simulink model "Demo_PreScanCarSim3D_ExtFMU_cs"  (Simulink 8.6)
settings: Solver=ode5  SolverMode=SingleTasking  StartTime=0.0  StopTime=68  FixedStep=1/1000  RelTol=1e-3
PreLoadFcn:
  | mbxruntime.callbacks.PreLoadFcn(bdroot);
  | check_NUTS_defined;
  | 
  | assignin('base',['model_closed_' bdroot],false);
PostLoadFcn:
  | mbxruntime.callbacks.PostLoadFcn(bdroot);
InitFcn:
  | mbxruntime.callbacks.InitFcn(bdroot);
StartFcn:
  | mbxruntime.callbacks.StartFcn(bdroot);
StopFcn:
  | mbxruntime.callbacks.StopFcn(bdroot);
undefined symbols (not defined in the file): DiscIntNeverNeededParam, mbxruntime, tabledata, warningInitialVelocity, x0, x_ini_VRML, y_ini_VRML, z_ini_VRML
libraries: PreScanSimulinkLibrary x15, simulink_extras x8, simulink x5, PreScanCarSimLibrary x1
(part 7 of 11)

== system Demo_PreScanCarSim3D_ExtFMU_cs/VISUMatrixSign_HighwayOverhang_1/ENABLED/Actuator ==
  VISUMatrixSign_HighwayOverhang_1 : Inport  Tag=inport/VisuMatrixSign  SampleTime=50/1000  BusOutputAsStruct=on
  DemuxVisuMatrixSign : Demux
  visu_MatrixSign_1 : S-Function  FunctionName=sfun_ResourceNameSelector  Parameters=mbxruntime.parameters.convert(UniqueID), mbxruntime.parameters.convert(ResourceList), mbxruntime.parameters.convert(PivotName),tabledata, TimeStep  SFunctionDeploymentMode=off  EnableBusSupport=off  mask(PreScan Sink Block: VisuMatrixSign){UniqueID=1876, ResourceList={'3' 'InformationSign\MatrixSign_Empty.png' '4' 'InformationSign\MatrixSign_End.png' '5' 'InformationSign\MatrixSign_GreenArrow.png' '6' 'InformationSign\MatrixSign_RedCross.png' '7' 'InformationSign\MatrixSign_Speed_50.png' '8' 'InformationSign\MatrixSign_Speed_70.png' '9' 'InformationSign\MatrixSign_Speed_90.png' '10' 'InformationSign\MatrixSign_Speed_120.png' '11' 'InformationSign\MatrixSign_Speed_130.png' '12' 'InformationSign\information.png' '13' 'InformationSign\TASS-international-logo.bmp' }, PivotName=/child:name=hcn/child:name=MatrixSign_1/trafficSignElement, TimeStep=50/1000}
      mask prompts: UniqueID "Parent Unique Identifier (auto-generated)"; ResourceList "Resource List (auto-generated)"; PivotName "Name of pivot (auto-generated)"; TimeStep "Simulink time step"
      mask help:
      | The VisuMatrixSign block provides a way to adapt the texture of the plates connected to an overhang, based on Resource IDs of the texture files.
      |
      | For more information, please click Help.
      mask init:
      | [tabledata] = mbxruntime.parameters.table(UniqueID,ResourceList,PivotName);
      mask Help: eval('openHelp(733)')
      mask Display: image(imread('HighwaySpeedMatrix.png'))
  visu_MatrixSign_2 : S-Function  FunctionName=sfun_ResourceNameSelector  Parameters=mbxruntime.parameters.convert(UniqueID), mbxruntime.parameters.convert(ResourceList), mbxruntime.parameters.convert(PivotName),tabledata, TimeStep  SFunctionDeploymentMode=off  EnableBusSupport=off  mask(PreScan Sink Block: VisuMatrixSign){UniqueID=1876, ResourceList={'3' 'InformationSign\MatrixSign_Empty.png' '4' 'InformationSign\MatrixSign_End.png' '5' 'InformationSign\MatrixSign_GreenArrow.png' '6' 'InformationSign\MatrixSign_RedCross.png' '7' 'InformationSign\MatrixSign_Speed_50.png' '8' 'InformationSign\MatrixSign_Speed_70.png' '9' 'InformationSign\MatrixSign_Speed_90.png' '10' 'InformationSign\MatrixSign_Speed_120.png' '11' 'InformationSign\MatrixSign_Speed_130.png' '12' 'InformationSign\information.png' '13' 'InformationSign\TASS-international-logo.bmp' }, PivotName=/child:name=hcn/child:name=MatrixSign_2/trafficSignElement, TimeStep=50/1000}
      mask prompts: UniqueID "Parent Unique Identifier (auto-generated)"; ResourceList "Resource List (auto-generated)"; PivotName "Name of pivot (auto-generated)"; TimeStep "Simulink time step"
      mask help:
      | The VisuMatrixSign block provides a way to adapt the texture of the plates connected to an overhang, based on Resource IDs of the texture files.
      |
      | For more information, please click Help.
      mask init:
      | [tabledata] = mbxruntime.parameters.table(UniqueID,ResourceList,PivotName);
      mask Help: eval('openHelp(733)')
      mask Display: image(imread('HighwaySpeedMatrix.png'))
  visu_MatrixSign_3 : S-Function  FunctionName=sfun_ResourceNameSelector  Parameters=mbxruntime.parameters.convert(UniqueID), mbxruntime.parameters.convert(ResourceList), mbxruntime.parameters.convert(PivotName),tabledata, TimeStep  SFunctionDeploymentMode=off  EnableBusSupport=off  mask(PreScan Sink Block: VisuMatrixSign){UniqueID=1876, ResourceList={'3' 'InformationSign\MatrixSign_Empty.png' '4' 'InformationSign\MatrixSign_End.png' '5' 'InformationSign\MatrixSign_GreenArrow.png' '6' 'InformationSign\MatrixSign_RedCross.png' '7' 'InformationSign\MatrixSign_Speed_50.png' '8' 'InformationSign\MatrixSign_Speed_70.png' '9' 'InformationSign\MatrixSign_Speed_90.png' '10' 'InformationSign\MatrixSign_Speed_120.png' '11' 'InformationSign\MatrixSign_Speed_130.png' '12' 'InformationSign\information.png' '13' 'InformationSign\TASS-international-logo.bmp' }, PivotName=/child:name=hcn/child:name=MatrixSign_3/trafficSignElement, TimeStep=50/1000}
      mask prompts: UniqueID "Parent Unique Identifier (auto-generated)"; ResourceList "Resource List (auto-generated)"; PivotName "Name of pivot (auto-generated)"; TimeStep "Simulink time step"
      mask help:
      | The VisuMatrixSign block provides a way to adapt the texture of the plates connected to an overhang, based on Resource IDs of the texture files.
      |
      | For more information, please click Help.
      mask init:
      | [tabledata] = mbxruntime.parameters.table(UniqueID,ResourceList,PivotName);
      mask Help: eval('openHelp(733)')
      mask Display: image(imread('HighwaySpeedMatrix.png'))
  visu_MatrixSign_4 : S-Function  FunctionName=sfun_ResourceNameSelector  Parameters=mbxruntime.parameters.convert(UniqueID), mbxruntime.parameters.convert(ResourceList), mbxruntime.parameters.convert(PivotName),tabledata, TimeStep  SFunctionDeploymentMode=off  EnableBusSupport=off  mask(PreScan Sink Block: VisuMatrixSign){UniqueID=1876, ResourceList={'3' 'InformationSign\MatrixSign_Empty.png' '4' 'InformationSign\MatrixSign_End.png' '5' 'InformationSign\MatrixSign_GreenArrow.png' '6' 'InformationSign\MatrixSign_RedCross.png' '7' 'InformationSign\MatrixSign_Speed_50.png' '8' 'InformationSign\MatrixSign_Speed_70.png' '9' 'InformationSign\MatrixSign_Speed_90.png' '10' 'InformationSign\MatrixSign_Speed_120.png' '11' 'InformationSign\MatrixSign_Speed_130.png' '12' 'InformationSign\information.png' '13' 'InformationSign\TASS-international-logo.bmp' }, PivotName=/child:name=hcn/child:name=MatrixSign_4/trafficSignElement, TimeStep=50/1000}
      mask prompts: UniqueID "Parent Unique Identifier (auto-generated)"; ResourceList "Resource List (auto-generated)"; PivotName "Name of pivot (auto-generated)"; TimeStep "Simulink time step"
      mask help:
      | The VisuMatrixSign block provides a way to adapt the texture of the plates connected to an overhang, based on Resource IDs of the texture files.
      |
      | For more information, please click Help.
      mask init:
      | [tabledata] = mbxruntime.parameters.table(UniqueID,ResourceList,PivotName);
      mask Help: eval('openHelp(733)')
      mask Display: image(imread('HighwaySpeedMatrix.png'))
  wires:
  VISUMatrixSign_HighwayOverhang_1/1 -> DemuxVisuMatrixSign/1
  DemuxVisuMatrixSign/1 -> visu_MatrixSign_1/1
  DemuxVisuMatrixSign/2 -> visu_MatrixSign_2/1
  DemuxVisuMatrixSign/3 -> visu_MatrixSign_3/1
  DemuxVisuMatrixSign/4 -> visu_MatrixSign_4/1

== system Demo_PreScanCarSim3D_ExtFMU_cs/VISUMatrixSign_HighwayOverhang_2/ENABLED/Actuator ==
  VISUMatrixSign_HighwayOverhang_2 : Inport  Tag=inport/VisuMatrixSign  SampleTime=50/1000  BusOutputAsStruct=on
  DemuxVisuMatrixSign : Demux  Outputs=3
  visu_MatrixSign_5 : S-Function  FunctionName=sfun_ResourceNameSelector  Parameters=mbxruntime.parameters.convert(UniqueID), mbxruntime.parameters.convert(ResourceList), mbxruntime.parameters.convert(PivotName),tabledata, TimeStep  SFunctionDeploymentMode=off  EnableBusSupport=off  mask(PreScan Sink Block: VisuMatrixSign){UniqueID=1877, ResourceList={'3' 'InformationSign\MatrixSign_Empty.png' '4' 'InformationSign\MatrixSign_End.png' '5' 'InformationSign\MatrixSign_GreenArrow.png' '6' 'InformationSign\MatrixSign_RedCross.png' '7' 'InformationSign\MatrixSign_Speed_50.png' '8' 'InformationSign\MatrixSign_Speed_70.png' '9' 'InformationSign\MatrixSign_Speed_90.png' '10' 'InformationSign\MatrixSign_Speed_120.png' '11' 'InformationSign\MatrixSign_Speed_130.png' '12' 'InformationSign\information.png' '13' 'InformationSign\TASS-international-logo.bmp' }, PivotName=/child:name=hcn/child:name=MatrixSign_5/trafficSignElement, TimeStep=50/1000}
      mask prompts: UniqueID "Parent Unique Identifier (auto-generated)"; ResourceList "Resource List (auto-generated)"; PivotName "Name of pivot (auto-generated)"; TimeStep "Simulink time step"
      mask help:
      | The VisuMatrixSign block provides a way to adapt the texture of the plates connected to an overhang, based on Resource IDs of the texture files.
      |
      | For more information, please click Help.
      mask init:
      | [tabledata] = mbxruntime.parameters.table(UniqueID,ResourceList,PivotName);
      mask Help: eval('openHelp(733)')
      mask Display: image(imread('HighwaySpeedMatrix.png'))
  visu_MatrixSign_6 : S-Function  FunctionName=sfun_ResourceNameSelector  Parameters=mbxruntime.parameters.convert(UniqueID), mbxruntime.parameters.convert(ResourceList), mbxruntime.parameters.convert(PivotName),tabledata, TimeStep  SFunctionDeploymentMode=off  EnableBusSupport=off  mask(PreScan Sink Block: VisuMatrixSign){UniqueID=1877, ResourceList={'3' 'InformationSign\MatrixSign_Empty.png' '4' 'InformationSign\MatrixSign_End.png' '5' 'InformationSign\MatrixSign_GreenArrow.png' '6' 'InformationSign\MatrixSign_RedCross.png' '7' 'InformationSign\MatrixSign_Speed_50.png' '8' 'InformationSign\MatrixSign_Speed_70.png' '9' 'InformationSign\MatrixSign_Speed_90.png' '10' 'InformationSign\MatrixSign_Speed_120.png' '11' 'InformationSign\MatrixSign_Speed_130.png' '12' 'InformationSign\information.png' '13' 'InformationSign\TASS-international-logo.bmp' }, PivotName=/child:name=hcn/child:name=MatrixSign_6/trafficSignElement, TimeStep=50/1000}
      mask prompts: UniqueID "Parent Unique Identifier (auto-generated)"; ResourceList "Resource List (auto-generated)"; PivotName "Name of pivot (auto-generated)"; TimeStep "Simulink time step"
      mask help:
      | The VisuMatrixSign block provides a way to adapt the texture of the plates connected to an overhang, based on Resource IDs of the texture files.
      |
      | For more information, please click Help.
      mask init:
      | [tabledata] = mbxruntime.parameters.table(UniqueID,ResourceList,PivotName);
      mask Help: eval('openHelp(733)')
      mask Display: image(imread('HighwaySpeedMatrix.png'))
  visu_MatrixSign_7 : S-Function  FunctionName=sfun_ResourceNameSelector  Parameters=mbxruntime.parameters.convert(UniqueID), mbxruntime.parameters.convert(ResourceList), mbxruntime.parameters.convert(PivotName),tabledata, TimeStep  SFunctionDeploymentMode=off  EnableBusSupport=off  mask(PreScan Sink Block: VisuMatrixSign){UniqueID=1877, ResourceList={'3' 'InformationSign\MatrixSign_Empty.png' '4' 'InformationSign\MatrixSign_End.png' '5' 'InformationSign\MatrixSign_GreenArrow.png' '6' 'InformationSign\MatrixSign_RedCross.png' '7' 'InformationSign\MatrixSign_Speed_50.png' '8' 'InformationSign\MatrixSign_Speed_70.png' '9' 'InformationSign\MatrixSign_Speed_90.png' '10' 'InformationSign\MatrixSign_Speed_120.png' '11' 'InformationSign\MatrixSign_Speed_130.png' '12' 'InformationSign\information.png' '13' 'InformationSign\TASS-international-logo.bmp' }, PivotName=/child:name=hcn/child:name=MatrixSign_7/trafficSignElement, TimeStep=50/1000}
      mask prompts: UniqueID "Parent Unique Identifier (auto-generated)"; ResourceList "Resource List (auto-generated)"; PivotName "Name of pivot (auto-generated)"; TimeStep "Simulink time step"
      mask help:
      | The VisuMatrixSign block provides a way to adapt the texture of the plates connected to an overhang, based on Resource IDs of the texture files.
      |
      | For more information, please click Help.
      mask init:
      | [tabledata] = mbxruntime.parameters.table(UniqueID,ResourceList,PivotName);
      mask Help: eval('openHelp(733)')
      mask Display: image(imread('HighwaySpeedMatrix.png'))
  wires:
  VISUMatrixSign_HighwayOverhang_2/1 -> DemuxVisuMatrixSign/1
  DemuxVisuMatrixSign/1 -> visu_MatrixSign_5/1
  DemuxVisuMatrixSign/2 -> visu_MatrixSign_6/1
  DemuxVisuMatrixSign/3 -> visu_MatrixSign_7/1

== system Demo_PreScanCarSim3D_ExtFMU_cs/VISUMatrixSign_HighwayOverhang_3/ENABLED/Actuator ==
  VISUMatrixSign_HighwayOverhang_3 : Inport  Tag=inport/VisuMatrixSign  SampleTime=50/1000  BusOutputAsStruct=on
  DemuxVisuMatrixSign : Demux  Outputs=3
  visu_MatrixSign_10 : S-Function  FunctionName=sfun_ResourceNameSelector  Parameters=mbxruntime.parameters.convert(UniqueID), mbxruntime.parameters.convert(ResourceList), mbxruntime.parameters.convert(PivotName),tabledata, TimeStep  SFunctionDeploymentMode=off  EnableBusSupport=off  mask(PreScan Sink Block: VisuMatrixSign){UniqueID=1890, ResourceList={'3' 'InformationSign\MatrixSign_Empty.png' '4' 'InformationSign\MatrixSign_End.png' '5' 'InformationSign\MatrixSign_GreenArrow.png' '6' 'InformationSign\MatrixSign_RedCross.png' '7' 'InformationSign\MatrixSign_Speed_50.png' '8' 'InformationSign\MatrixSign_Speed_70.png' '9' 'InformationSign\MatrixSign_Speed_90.png' '10' 'InformationSign\MatrixSign_Speed_120.png' '11' 'InformationSign\MatrixSign_Speed_130.png' '12' 'InformationSign\information.png' '13' 'InformationSign\TASS-international-logo.bmp' }, PivotName=/child:name=hcn/child:name=MatrixSign_10/trafficSignElement, TimeStep=50/1000}
      mask prompts: UniqueID "Parent Unique Identifier (auto-generated)"; ResourceList "Resource List (auto-generated)"; PivotName "Name of pivot (auto-generated)"; TimeStep "Simulink time step"
      mask help:
      | The VisuMatrixSign block provides a way to adapt the texture of the plates connected to an overhang, based on Resource IDs of the texture files.
      |
      | For more information, please click Help.
      mask init:
      | [tabledata] = mbxruntime.parameters.table(UniqueID,ResourceList,PivotName);
      mask Help: eval('openHelp(733)')
      mask Display: image(imread('HighwaySpeedMatrix.png'))
  visu_MatrixSign_11 : S-Function  FunctionName=sfun_ResourceNameSelector  Parameters=mbxruntime.parameters.convert(UniqueID), mbxruntime.parameters.convert(ResourceList), mbxruntime.parameters.convert(PivotName),tabledata, TimeStep  SFunctionDeploymentMode=off  EnableBusSupport=off  mask(PreScan Sink Block: VisuMatrixSign){UniqueID=1890, ResourceList={'3' 'InformationSign\MatrixSign_Empty.png' '4' 'InformationSign\MatrixSign_End.png' '5' 'InformationSign\MatrixSign_GreenArrow.png' '6' 'InformationSign\MatrixSign_RedCross.png' '7' 'InformationSign\MatrixSign_Speed_50.png' '8' 'InformationSign\MatrixSign_Speed_70.png' '9' 'InformationSign\MatrixSign_Speed_90.png' '10' 'InformationSign\MatrixSign_Speed_120.png' '11' 'InformationSign\MatrixSign_Speed_130.png' '12' 'InformationSign\information.png' '13' 'InformationSign\TASS-international-logo.bmp' }, PivotName=/child:name=hcn/child:name=MatrixSign_11/trafficSignElement, TimeStep=50/1000}
      mask prompts: UniqueID "Parent Unique Identifier (auto-generated)"; ResourceList "Resource List (auto-generated)"; PivotName "Name of pivot (auto-generated)"; TimeStep "Simulink time step"
      mask help:
      | The VisuMatrixSign block provides a way to adapt the texture of the plates connected to an overhang, based on Resource IDs of the texture files.
      |
      | For more information, please click Help.
      mask init:
      | [tabledata] = mbxruntime.parameters.table(UniqueID,ResourceList,PivotName);
      mask Help: eval('openHelp(733)')
      mask Display: image(imread('HighwaySpeedMatrix.png'))
  visu_MatrixSign_12 : S-Function  FunctionName=sfun_ResourceNameSelector  Parameters=mbxruntime.parameters.convert(UniqueID), mbxruntime.parameters.convert(ResourceList), mbxruntime.parameters.convert(PivotName),tabledata, TimeStep  SFunctionDeploymentMode=off  EnableBusSupport=off  mask(PreScan Sink Block: VisuMatrixSign){UniqueID=1890, ResourceList={'3' 'InformationSign\MatrixSign_Empty.png' '4' 'InformationSign\MatrixSign_End.png' '5' 'InformationSign\MatrixSign_GreenArrow.png' '6' 'InformationSign\MatrixSign_RedCross.png' '7' 'InformationSign\MatrixSign_Speed_50.png' '8' 'InformationSign\MatrixSign_Speed_70.png' '9' 'InformationSign\MatrixSign_Speed_90.png' '10' 'InformationSign\MatrixSign_Speed_120.png' '11' 'InformationSign\MatrixSign_Speed_130.png' '12' 'InformationSign\information.png' '13' 'InformationSign\TASS-international-logo.bmp' }, PivotName=/child:name=hcn/child:name=MatrixSign_12/trafficSignElement, TimeStep=50/1000}
      mask prompts: UniqueID "Parent Unique Identifier (auto-generated)"; ResourceList "Resource List (auto-generated)"; PivotName "Name of pivot (auto-generated)"; TimeStep "Simulink time step"
      mask help:
      | The VisuMatrixSign block provides a way to adapt the texture of the plates connected to an overhang, based on Resource IDs of the texture files.
      |
      | For more information, please click Help.
      mask init:
      | [tabledata] = mbxruntime.parameters.table(UniqueID,ResourceList,PivotName);
      mask Help: eval('openHelp(733)')
      mask Display: image(imread('HighwaySpeedMatrix.png'))
  wires:
  VISUMatrixSign_HighwayOverhang_3/1 -> DemuxVisuMatrixSign/1
  DemuxVisuMatrixSign/1 -> visu_MatrixSign_10/1
  DemuxVisuMatrixSign/2 -> visu_MatrixSign_11/1
  DemuxVisuMatrixSign/3 -> visu_MatrixSign_12/1

== system Demo_PreScanCarSim3D_ExtFMU_cs/VISUMatrixSign_HighwayOverhang_5/ENABLED/Actuator ==
  VISUMatrixSign_HighwayOverhang_5 : Inport  Tag=inport/VisuMatrixSign  SampleTime=50/1000  BusOutputAsStruct=on
  DemuxVisuMatrixSign : Demux  Outputs=3
  visu_MatrixSign_18 : S-Function  FunctionName=sfun_ResourceNameSelector  Parameters=mbxruntime.parameters.convert(UniqueID), mbxruntime.parameters.convert(ResourceList), mbxruntime.parameters.convert(PivotName),tabledata, TimeStep  SFunctionDeploymentMode=off  EnableBusSupport=off  mask(PreScan Sink Block: VisuMatrixSign){UniqueID=1909, ResourceList={'3' 'InformationSign\MatrixSign_Empty.png' '4' 'InformationSign\MatrixSign_End.png' '5' 'InformationSign\MatrixSign_GreenArrow.png' '6' 'InformationSign\MatrixSign_RedCross.png' '7' 'InformationSign\MatrixSign_Speed_50.png' '8' 'InformationSign\MatrixSign_Speed_70.png' '9' 'InformationSign\MatrixSign_Speed_90.png' '10' 'InformationSign\MatrixSign_Speed_120.png' '11' 'InformationSign\MatrixSign_Speed_130.png' '12' 'InformationSign\information.png' '13' 'InformationSign\TASS-international-logo.bmp' }, PivotName=/child:name=hcn/child:name=MatrixSign_18/trafficSignElement, TimeStep=50/1000}
      mask prompts: UniqueID "Parent Unique Identifier (auto-generated)"; ResourceList "Resource List (auto-generated)"; PivotName "Name of pivot (auto-generated)"; TimeStep "Simulink time step"
      mask help:
      | The VisuMatrixSign block provides a way to adapt the texture of the plates connected to an overhang, based on Resource IDs of the texture files.
      |
      | For more information, please click Help.
      mask init:
      | [tabledata] = mbxruntime.parameters.table(UniqueID,ResourceList,PivotName);
      mask Help: eval('openHelp(733)')
      mask Display: image(imread('HighwaySpeedMatrix.png'))
  visu_MatrixSign_19 : S-Function  FunctionName=sfun_ResourceNameSelector  Parameters=mbxruntime.parameters.convert(UniqueID), mbxruntime.parameters.convert(ResourceList), mbxruntime.parameters.convert(PivotName),tabledata, TimeStep  SFunctionDeploymentMode=off  EnableBusSupport=off  mask(PreScan Sink Block: VisuMatrixSign){UniqueID=1909, ResourceList={'3' 'InformationSign\MatrixSign_Empty.png' '4' 'InformationSign\MatrixSign_End.png' '5' 'InformationSign\MatrixSign_GreenArrow.png' '6' 'InformationSign\MatrixSign_RedCross.png' '7' 'InformationSign\MatrixSign_Speed_50.png' '8' 'InformationSign\MatrixSign_Speed_70.png' '9' 'InformationSign\MatrixSign_Speed_90.png' '10' 'InformationSign\MatrixSign_Speed_120.png' '11' 'InformationSign\MatrixSign_Speed_130.png' '12' 'InformationSign\information.png' '13' 'InformationSign\TASS-international-logo.bmp' }, PivotName=/child:name=hcn/child:name=MatrixSign_19/trafficSignElement, TimeStep=50/1000}
      mask prompts: UniqueID "Parent Unique Identifier (auto-generated)"; ResourceList "Resource List (auto-generated)"; PivotName "Name of pivot (auto-generated)"; TimeStep "Simulink time step"
      mask help:
      | The VisuMatrixSign block provides a way to adapt the texture of the plates connected to an overhang, based on Resource IDs of the texture files.
      |
      | For more information, please click Help.
      mask init:
      | [tabledata] = mbxruntime.parameters.table(UniqueID,ResourceList,PivotName);
      mask Help: eval('openHelp(733)')
      mask Display: image(imread('HighwaySpeedMatrix.png'))
  visu_MatrixSign_20 : S-Function  FunctionName=sfun_ResourceNameSelector  Parameters=mbxruntime.parameters.convert(UniqueID), mbxruntime.parameters.convert(ResourceList), mbxruntime.parameters.convert(PivotName),tabledata, TimeStep  SFunctionDeploymentMode=off  EnableBusSupport=off  mask(PreScan Sink Block: VisuMatrixSign){UniqueID=1909, ResourceList={'3' 'InformationSign\MatrixSign_Empty.png' '4' 'InformationSign\MatrixSign_End.png' '5' 'InformationSign\MatrixSign_GreenArrow.png' '6' 'InformationSign\MatrixSign_RedCross.png' '7' 'InformationSign\MatrixSign_Speed_50.png' '8' 'InformationSign\MatrixSign_Speed_70.png' '9' 'InformationSign\MatrixSign_Speed_90.png' '10' 'InformationSign\MatrixSign_Speed_120.png' '11' 'InformationSign\MatrixSign_Speed_130.png' '12' 'InformationSign\information.png' '13' 'InformationSign\TASS-international-logo.bmp' }, PivotName=/child:name=hcn/child:name=MatrixSign_20/trafficSignElement, TimeStep=50/1000}
      mask prompts: UniqueID "Parent Unique Identifier (auto-generated)"; ResourceList "Resource List (auto-generated)"; PivotName "Name of pivot (auto-generated)"; TimeStep "Simulink time step"
      mask help:
      | The VisuMatrixSign block provides a way to adapt the texture of the plates connected to an overhang, based on Resource IDs of the texture files.
      |
      | For more information, please click Help.
      mask init:
      | [tabledata] = mbxruntime.parameters.table(UniqueID,ResourceList,PivotName);
      mask Help: eval('openHelp(733)')
      mask Display: image(imread('HighwaySpeedMatrix.png'))
  wires:
  VISUMatrixSign_HighwayOverhang_5/1 -> DemuxVisuMatrixSign/1
  DemuxVisuMatrixSign/1 -> visu_MatrixSign_18/1
  DemuxVisuMatrixSign/2 -> visu_MatrixSign_19/1
  DemuxVisuMatrixSign/3 -> visu_MatrixSign_20/1

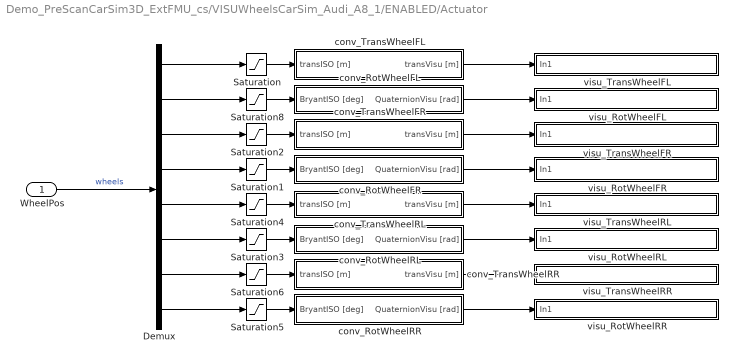
== system Demo_PreScanCarSim3D_ExtFMU_cs/VISUWheelsCarSim_Audi_A8_1/ENABLED/Actuator ==
  WheelPos : Inport
  Demux : Demux  Outputs=[3 3 3 3 3 3 3 3]
  Saturation{,2,4,6} (4 alike) : Saturate  UpperLimit=[0.2 0.2 0.5]  LowerLimit=[-0.2 -0.2 -0.5]
  Saturation{1,3,5,8} (4 alike) : Saturate  UpperLimit=[30 inf 30]  LowerLimit=[-30 -inf -30]
  conv_RotWheelFL : Subsystem
  conv_RotWheelFR : Subsystem
  conv_RotWheelRL : Subsystem
  conv_RotWheelRR : Subsystem
  conv_TransWheelFL : Subsystem  mask(Translation node configuration){tp=Front-Left Wheel, gains=off, Gain_xISO=1, Gain_yISO=1, Gain_zISO=1}
      mask prompts: tp "Type"; gains "Edit scaling factors?"; Gain_xISO "Scaling factor in x-direction (ISO-convention)"; Gain_yISO "Scaling factor in y-direction (ISO-convention)"; Gain_zISO "Scaling factor in z-direction (ISO-convention)"
      mask init:
      | [x_ini_VRML,y_ini_VRML,z_ini_VRML]=Visu_ini_param('Audi_A8',tp);
      mask TypeOptions tp: Front-Left Wheel | Front-Right Wheel | Rear-Left Wheel | Rear-Right Wheel | Left Seat | Right Seat
      mask Callback gains:
      | if strcmp(get_param(gcb, 'gains'),'on')
      |     set_param(gcb,'MaskVisibilities',{'on','on','on','on','on'})
      | else
      |     set_param(gcb,'MaskVisibilities',{'on','on','off','off','off'})
      | end
  conv_TransWheelFR : Subsystem  mask(Translation node configuration){tp=Front-Right Wheel, gains=off, Gain_xISO=1, Gain_yISO=1, Gain_zISO=1}
      mask prompts: tp "Type"; gains "Edit scaling factors?"; Gain_xISO "Scaling factor in x-direction (ISO-convention)"; Gain_yISO "Scaling factor in y-direction (ISO-convention)"; Gain_zISO "Scaling factor in z-direction (ISO-convention)"
      mask init:
      | [x_ini_VRML,y_ini_VRML,z_ini_VRML]=Visu_ini_param('Audi_A8',tp);
      mask TypeOptions tp: Front-Left Wheel | Front-Right Wheel | Rear-Left Wheel | Rear-Right Wheel | Left Seat | Right Seat
      mask Callback gains:
      | if strcmp(get_param(gcb, 'gains'),'on')
      |     set_param(gcb,'MaskVisibilities',{'on','on','on','on','on'})
      | else
      |     set_param(gcb,'MaskVisibilities',{'on','on','off','off','off'})
      | end
  conv_TransWheelRL : Subsystem  mask(Translation node configuration){tp=Rear-Left Wheel, gains=off, Gain_xISO=1, Gain_yISO=1, Gain_zISO=1}
      mask prompts: tp "Type"; gains "Edit scaling factors?"; Gain_xISO "Scaling factor in x-direction (ISO-convention)"; Gain_yISO "Scaling factor in y-direction (ISO-convention)"; Gain_zISO "Scaling factor in z-direction (ISO-convention)"
      mask init:
      | [x_ini_VRML,y_ini_VRML,z_ini_VRML]=Visu_ini_param('Audi_A8',tp);
      mask TypeOptions tp: Front-Left Wheel | Front-Right Wheel | Rear-Left Wheel | Rear-Right Wheel | Left Seat | Right Seat
      mask Callback gains:
      | if strcmp(get_param(gcb, 'gains'),'on')
      |     set_param(gcb,'MaskVisibilities',{'on','on','on','on','on'})
      | else
      |     set_param(gcb,'MaskVisibilities',{'on','on','off','off','off'})
      | end
  conv_TransWheelRR : Subsystem  mask(Translation node configuration){tp=Rear-Right Wheel, gains=off, Gain_xISO=1, Gain_yISO=1, Gain_zISO=1}
      mask prompts: tp "Type"; gains "Edit scaling factors?"; Gain_xISO "Scaling factor in x-direction (ISO-convention)"; Gain_yISO "Scaling factor in y-direction (ISO-convention)"; Gain_zISO "Scaling factor in z-direction (ISO-convention)"
      mask init:
      | [x_ini_VRML,y_ini_VRML,z_ini_VRML]=Visu_ini_param('Audi_A8',tp);
      mask TypeOptions tp: Front-Left Wheel | Front-Right Wheel | Rear-Left Wheel | Rear-Right Wheel | Left Seat | Right Seat
      mask Callback gains:
      | if strcmp(get_param(gcb, 'gains'),'on')
      |     set_param(gcb,'MaskVisibilities',{'on','on','on','on','on'})
      | else
      |     set_param(gcb,'MaskVisibilities',{'on','on','off','off','off'})
      | end
  visu_RotWheelFL : Subsystem  mask(AxisAngleActuator){UniqueID=UniqueID, Object3DID=[ObjectName '.WheelFL'], TimeStep=TimeStep}
      mask prompts: UniqueID "Auto-Assigned: Unique ID"; Object3DID "Auto-Assigned: Child 3D Object ID"; TimeStep "Auto-Assigned: Upload Period [s]"
      mask help: Applies axis angle update to selected child object
      mask Help:
      | Applies axis angle update to selected child object
      | 
      | - UniqueID (double)   : Unique ID of the parent actor
      | - Object3DID (string) : Name of the child 3D object
      mask Display: port_label('input', 1, ['AxisAngle ' Object3DID])
  visu_RotWheelFR : Subsystem  mask(AxisAngleActuator){UniqueID=UniqueID, Object3DID=[ObjectName '.WheelFR'], TimeStep=TimeStep}
      mask prompts: UniqueID "Auto-Assigned: Unique ID"; Object3DID "Auto-Assigned: Child 3D Object ID"; TimeStep "Auto-Assigned: Upload Period [s]"
      mask help: Applies axis angle update to selected child object
      mask Help:
      | Applies axis angle update to selected child object
      | 
      | - UniqueID (double)   : Unique ID of the parent actor
      | - Object3DID (string) : Name of the child 3D object
      mask Display: port_label('input', 1, ['AxisAngle ' Object3DID])
  visu_RotWheelRL : Subsystem  mask(AxisAngleActuator){UniqueID=UniqueID, Object3DID=[ObjectName '.WheelRL'], TimeStep=TimeStep}
      mask prompts: UniqueID "Auto-Assigned: Unique ID"; Object3DID "Auto-Assigned: Child 3D Object ID"; TimeStep "Auto-Assigned: Upload Period [s]"
      mask help: Applies axis angle update to selected child object
      mask Help:
      | Applies axis angle update to selected child object
      | 
      | - UniqueID (double)   : Unique ID of the parent actor
      | - Object3DID (string) : Name of the child 3D object
      mask Display: port_label('input', 1, ['AxisAngle ' Object3DID])
  visu_RotWheelRR : Subsystem  mask(AxisAngleActuator){UniqueID=UniqueID, Object3DID=[ObjectName '.WheelRR'], TimeStep=TimeStep}
      mask prompts: UniqueID "Auto-Assigned: Unique ID"; Object3DID "Auto-Assigned: Child 3D Object ID"; TimeStep "Auto-Assigned: Upload Period [s]"
      mask help: Applies axis angle update to selected child object
      mask Help:
      | Applies axis angle update to selected child object
      | 
      | - UniqueID (double)   : Unique ID of the parent actor
      | - Object3DID (string) : Name of the child 3D object
      mask Display: port_label('input', 1, ['AxisAngle ' Object3DID])
  visu_TransWheelFL : Subsystem  mask(PositionActuator){UniqueID=UniqueID, Object3DID=[ObjectName '.WheelFL'], TimeStep=TimeStep}
      mask prompts: UniqueID "Auto-Assigned: Unique ID"; Object3DID "Auto-Assigned: Child 3D Object ID"; TimeStep "Auto-Assigned: Upload Period [s]"
      mask help: Applies position update to selected child object
      mask Help:
      | Applies position update to selected child object
      | 
      | - UniqueID (double)   : Unique ID of the parent actor
      | - Object3DID (string) : Name of the child 3D object
      mask Display: port_label('input', 1, ['Position ' Object3DID])
  visu_TransWheelFR : Subsystem  mask(PositionActuator){UniqueID=UniqueID, Object3DID=[ObjectName '.WheelFR'], TimeStep=TimeStep}
      mask prompts: UniqueID "Auto-Assigned: Unique ID"; Object3DID "Auto-Assigned: Child 3D Object ID"; TimeStep "Auto-Assigned: Upload Period [s]"
      mask help: Applies position update to selected child object
      mask Help:
      | Applies position update to selected child object
      | 
      | - UniqueID (double)   : Unique ID of the parent actor
      | - Object3DID (string) : Name of the child 3D object
      mask Display: port_label('input', 1, ['Position ' Object3DID])
  visu_TransWheelRL : Subsystem  mask(PositionActuator){UniqueID=UniqueID, Object3DID=[ObjectName '.WheelRL'], TimeStep=TimeStep}
      mask prompts: UniqueID "Auto-Assigned: Unique ID"; Object3DID "Auto-Assigned: Child 3D Object ID"; TimeStep "Auto-Assigned: Upload Period [s]"
      mask help: Applies position update to selected child object
      mask Help:
      | Applies position update to selected child object
      | 
      | - UniqueID (double)   : Unique ID of the parent actor
      | - Object3DID (string) : Name of the child 3D object
      mask Display: port_label('input', 1, ['Position ' Object3DID])
  visu_TransWheelRR : Subsystem  mask(PositionActuator){UniqueID=UniqueID, Object3DID=[ObjectName '.WheelRR'], TimeStep=TimeStep}
      mask prompts: UniqueID "Auto-Assigned: Unique ID"; Object3DID "Auto-Assigned: Child 3D Object ID"; TimeStep "Auto-Assigned: Upload Period [s]"
      mask help: Applies position update to selected child object
      mask Help:
      | Applies position update to selected child object
      | 
      | - UniqueID (double)   : Unique ID of the parent actor
      | - Object3DID (string) : Name of the child 3D object
      mask Display: port_label('input', 1, ['Position ' Object3DID])
  wires:
  WheelPos/1 -> Demux/1  "wheels"
  conv_RotWheelRR/1(QuaternionVisu [rad]) -> visu_RotWheelRR/1(In1)
  conv_RotWheelRL/1(QuaternionVisu [rad]) -> visu_RotWheelRL/1(In1)
  conv_RotWheelFR/1(QuaternionVisu [rad]) -> visu_RotWheelFR/1(In1)
  conv_TransWheelRR/1(transVisu [m]) -> visu_TransWheelRR/1(In1)
  conv_TransWheelRL/1(transVisu [m]) -> visu_TransWheelRL/1(In1)
  conv_TransWheelFR/1(transVisu [m]) -> visu_TransWheelFR/1(In1)
  Saturation/1 -> conv_TransWheelFL/1(transISO [m])
  Saturation8/1 -> conv_RotWheelFL/1(BryantISO [deg])
  Saturation2/1 -> conv_TransWheelFR/1(transISO [m])
  Saturation1/1 -> conv_RotWheelFR/1(BryantISO [deg])
  Saturation4/1 -> conv_TransWheelRL/1(transISO [m])
  Saturation3/1 -> conv_RotWheelRL/1(BryantISO [deg])
  Saturation6/1 -> conv_TransWheelRR/1(transISO [m])
  Saturation5/1 -> conv_RotWheelRR/1(BryantISO [deg])
  Demux/1 -> Saturation/1
  Demux/2 -> Saturation8/1
  Demux/3 -> Saturation2/1
  Demux/4 -> Saturation1/1
  Demux/5 -> Saturation4/1
  Demux/6 -> Saturation3/1
  Demux/7 -> Saturation6/1
  Demux/8 -> Saturation5/1
  conv_TransWheelFL/1(transVisu [m]) -> visu_TransWheelFL/1(In1)
  conv_RotWheelFL/1(QuaternionVisu [rad]) -> visu_RotWheelFL/1(In1)

== system Demo_PreScanCarSim3D_ExtFMU_cs/Audi_A8_1/ENABLED/CarSim_Vehicle/CarSim2PreScanSTATE ==
  CarSim_In : Inport
  D2R : Gain  Gain=pi/180
  Demux : Demux  Outputs=[3 3 3 -1]
  Demux1 : Demux  Outputs=3
  Demux2 : Demux  Outputs=3
  Demux3 : Demux  Outputs=3
  Terminator : Terminator
  Transformation_SprungMassCarSim2PreScan : Subsystem
  km|h_to_m|s : Gain  Gain=1/3.6
  x [m] : Outport
  y [m] : Outport  Port=2
  z [m] : Outport  Port=3
  dx [m/s] : Outport  Port=4
  dy [m/s] : Outport  Port=5
  dz [m/s] : Outport  Port=6
  R [rad] : Outport  Port=7
  P [rad] : Outport  Port=8
  Y [rad] : Outport  Port=9
  wires:
  Demux/4 -> Terminator/1
  Demux3/3 -> Y [rad]/1
  Demux3/2 -> P [rad]/1
  Demux3/1 -> R [rad]/1
  Demux2/3 -> dz [m/s]/1
  Demux2/2 -> dy [m/s]/1
  Demux2/1 -> dx [m/s]/1
  Demux1/3 -> z [m]/1
  Demux1/2 -> y [m]/1
  Demux1/1 -> x [m]/1
  Transformation_SprungMassCarSim2PreScan/1(Out1) -> Demux1/1
  Demux/1 -> Transformation_SprungMassCarSim2PreScan/1(In1)
  CarSim_In/1 -> Demux/1
  km|h_to_m|s/1 -> Demux2/1
  Demux/2 -> km|h_to_m|s/1
  Demux/3 -> D2R/1
  D2R/1 -> Demux3/1

== system Demo_PreScanCarSim3D_ExtFMU_cs/Audi_A8_1/ENABLED/CarSim_Vehicle/CarSim2PreScan_BUS ==
  CarSim_In : Inport
  Bus Creator2 : BusCreator  Inputs=3
  Bus Creator9 : BusCreator  Inputs=1
  Demux : Demux  Outputs=[3 3 3 12 12 2]
  Steering : Subsystem
  Vehicle : Subsystem
  Wheel : Subsystem
  PreScanBUS_VehicleDynamics : Outport
  wires:
  Steering/1(Steering) -> Bus Creator2/3
  Demux/6 -> Steering/1(SteeringWheel_In)  "SteeringWheel_In"
  CarSim_In/1 -> Demux/1
  Demux/1 -> Wheel/1(SprungMass_Pos_Global[x;y;z][m])  "SprungMass_Pos_Global[x;y;z][m]"
  Demux/5 -> Wheel/4(CarSim_Angle_Wheel_[FL;FR;RL;RR][x;y;z][deg;rev;deg])  "CarSim_Angle_Wheel_[FL;FR;RL;RR][x;y;z][deg;rev;deg]"
  Demux/4 -> Wheel/3(CarSim_Pos_Wheel_[FL;FR;RL;RR][x;y;z][m])  "CarSim_Pos_Wheel_[FL;FR;RL;RR][x;y;z][m]"
  Demux/3 -> Wheel/2(SprungMass_Angle_Global[x;y;z][deg])  "SprungMass_Angle_Global[x;y;z][deg]"
  Demux/2 -> Vehicle/1(v_VehicleCoG[x;y;z][km|h])  "v_VehicleCoG[x;y;z][km|h]"
  Wheel/1(Wheel) -> Bus Creator2/2
  Vehicle/1(Vehicle) -> Bus Creator2/1
  Bus Creator9/1 -> PreScanBUS_VehicleDynamics/1
  Bus Creator2/1 -> Bus Creator9/1  "PreScanBUS_VehicleDynamics"

== system Demo_PreScanCarSim3D_ExtFMU_cs/Audi_A8_1/ENABLED/CarSim_Vehicle/CarSim2PreScan_ContactAdapter ==
  State : Inport
  State_Bus : Inport  Port=2
  Bus Selector : BusSelector  OutputSignals=PreScanBUS_VehicleDynamics.Vehicle.Velocities.Linear,PreScanBUS_VehicleDynamics.Wheel.Position.Linear
  Constant : Constant  Value=[ wheelRadius wheelRadius wheelRadius wheelRadius ]
  Embedded MATLAB Function : MATLAB Function  TreatAsAtomicUnit=on
  Memory : Memory
  Mux : Mux  Inputs="[9 1 12  4]"
  ContactParams : Outport
  wires:
  Memory/1 -> ContactParams/1
  Constant/1 -> Mux/4
  Bus Selector/1 -> Embedded MATLAB Function/1(u)  "<Linear>"
  State_Bus/1 -> Bus Selector/1
  Bus Selector/2 -> Mux/3  "<Linear>"
  State/1 -> Mux/1
  Embedded MATLAB Function/1(y) -> Mux/2
  Mux/1 -> Memory/1

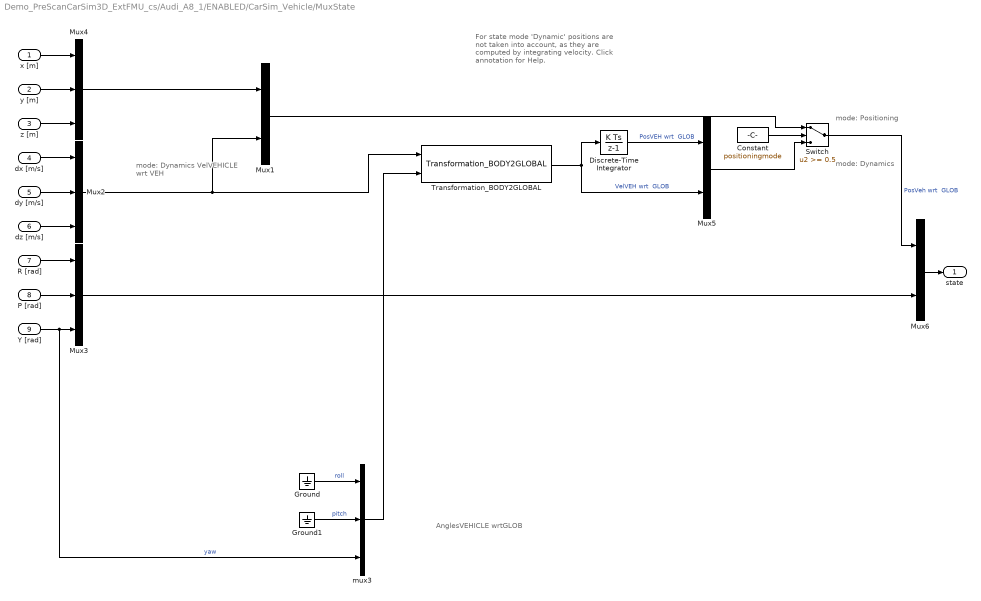
== system Demo_PreScanCarSim3D_ExtFMU_cs/Audi_A8_1/ENABLED/CarSim_Vehicle/MuxState ==
  note: mode: Dynamics
  note: mode: Positioning
  note: mode: Dynamics
      | VelVEHICLE
      | wrt VEH
  note: AnglesVEHICLE
      | wrtGLOB
  note: For state mode 'Dynamic' positions
      | are not taken into account, as they
      | are computed by integrating velocity.
      | Click annotation for Help.
  x [m] : Inport  SampleTime=TimeStep
  y [m] : Inport  Port=2  SampleTime=TimeStep
  z [m] : Inport  Port=3  SampleTime=TimeStep
  dx [m/s] : Inport  Port=4  SampleTime=TimeStep
  dy [m/s] : Inport  Port=5  SampleTime=TimeStep
  dz [m/s] : Inport  Port=6  SampleTime=TimeStep
  R [rad] : Inport  Port=7  SampleTime=TimeStep
  P [rad] : Inport  Port=8  SampleTime=TimeStep
  Y [rad] : Inport  Port=9  SampleTime=TimeStep
  Constant : Constant  DisableCoverage=on  Value=positioningmode
  Discrete-Time Integrator : DiscreteIntegrator  SampleTime=TimeStep  ICPrevOutput=DiscIntNeverNeededParam  ICPrevScaledInput=DiscIntNeverNeededParam
  Ground : Ground
  Ground1 : Ground
  Mux1 : Mux  Inputs=[3 3]
  Mux2 : Mux  Inputs=3
  Mux3 : Mux  Inputs=3
  Mux4 : Mux  Inputs=3
  Mux5 : Mux  Inputs=[3 3]
  Mux6 : Mux  Inputs=[6 3]
  Switch : Switch  Threshold=0.5
  Transformation_BODY2GLOBAL : PreScanSimulinkLibrary/Simple_Vehicle_Dynamics/Chassis/MuxDynState/Transformation_BODY2GLOBAL
  mux3 : Mux  Inputs=3
  state : Outport
  wires:
  Constant/1 -> Switch/2
  Mux6/1 -> state/1
  Mux4/1 -> Mux1/1
  Mux5/1 -> Switch/3
  Mux1/1 -> Switch/1
  Switch/1 -> Mux6/1  "PosVeh wrt  GLOB"
  P [rad]/1 -> Mux3/2
  R [rad]/1 -> Mux3/1
  dz [m/s]/1 -> Mux2/3
  dy [m/s]/1 -> Mux2/2
  dx [m/s]/1 -> Mux2/1
  z [m]/1 -> Mux4/3
  y [m]/1 -> Mux4/2
  x [m]/1 -> Mux4/1
  Ground1/1 -> mux3/2  "pitch"
  Y [rad]/1 -> mux3/3, Mux3/3  "yaw"
  Mux3/1 -> Mux6/2
  Transformation_BODY2GLOBAL/1 -> Discrete-Time Integrator/1, Mux5/2  "VelVEH wrt  GLOB"
  mux3/1 -> Transformation_BODY2GLOBAL/2
  Ground/1 -> mux3/1  "roll"
  Mux2/1 -> Mux1/2, Transformation_BODY2GLOBAL/1
  Discrete-Time Integrator/1 -> Mux5/1  "PosVEH wrt  GLOB"

== system Demo_PreScanCarSim3D_ExtFMU_cs/Audi_A8_1/ENABLED/CarSim_Vehicle/TyreContact To Road Information ==
  TyreInfo_in : Inport
  Bus Selector3 : BusSelector  OutputSignals=TireFL.normal.x,TireFL.normal.y,TireFL.normal.z,TireFL.position.z,TireFR.normal.x,TireFR.normal.y,TireFR.normal.z,TireFR.position.z,TireRL.normal.x,TireRL.normal.y,TireRL.normal.z,TireRL.position.z,TireRR.normal.x,TireRR.normal.y,TireRR.normal.z,TireRR.position.z
  Contact To Road Information : Subsystem
  RoadSlopeAndZ_[FL;FR;RL;RR] : Outport
  wires:
  Bus Selector3/8 -> Contact To Road Information/8(" Pos_z_CP_CoorSys_E[FR]m]")  "<z>"
  Bus Selector3/7 -> Contact To Road Information/7(UnitVec_z_CP_CoorSys_E[FR][z])  "<z>"
  Contact To Road Information/1(RoadSlopeAndZ_[FL;FR;RL;RR]) -> RoadSlopeAndZ_[FL;FR;RL;RR]/1
  Bus Selector3/16 -> Contact To Road Information/16(" Pos_z_CP_CoorSys_E[RR]m]")  "<z>"
  Bus Selector3/15 -> Contact To Road Information/15(UnitVec_z_CP_CoorSys_E[RR][z])  "<z>"
  Bus Selector3/14 -> Contact To Road Information/14(UnitVec_z_CP_CoorSys_E[RR][y])  "<y>"
  Bus Selector3/13 -> Contact To Road Information/13(UnitVec_z_CP_CoorSys_E[RR][x])  "<x>"
  Bus Selector3/12 -> Contact To Road Information/12(" Pos_z_CP_CoorSys_E[RL]m]")  "<z>"
  Bus Selector3/11 -> Contact To Road Information/11(UnitVec_z_CP_CoorSys_E[RL][z])  "<z>"
  Bus Selector3/10 -> Contact To Road Information/10(UnitVec_z_CP_CoorSys_E[RL][y])  "<y>"
  Bus Selector3/9 -> Contact To Road Information/9(UnitVec_z_CP_CoorSys_E[RL][x])  "<x>"
  Bus Selector3/6 -> Contact To Road Information/6(UnitVec_z_CP_CoorSys_E[FR][y])  "<y>"
  Bus Selector3/5 -> Contact To Road Information/5(UnitVec_z_CP_CoorSys_E[FR][x])  "<x>"
  Bus Selector3/4 -> Contact To Road Information/4(" Pos_z_CP_CoorSys_E[FL]m]")  "<z>"
  Bus Selector3/3 -> Contact To Road Information/3(UnitVec_z_CP_CoorSys_E[FL][z])  "<z>"
  Bus Selector3/2 -> Contact To Road Information/2(UnitVec_z_CP_CoorSys_E[FL][y])  "<y>"
  Bus Selector3/1 -> Contact To Road Information/1(UnitVec_z_CP_CoorSys_E[FL][x])  "<x>"
  TyreInfo_in/1 -> Bus Selector3/1

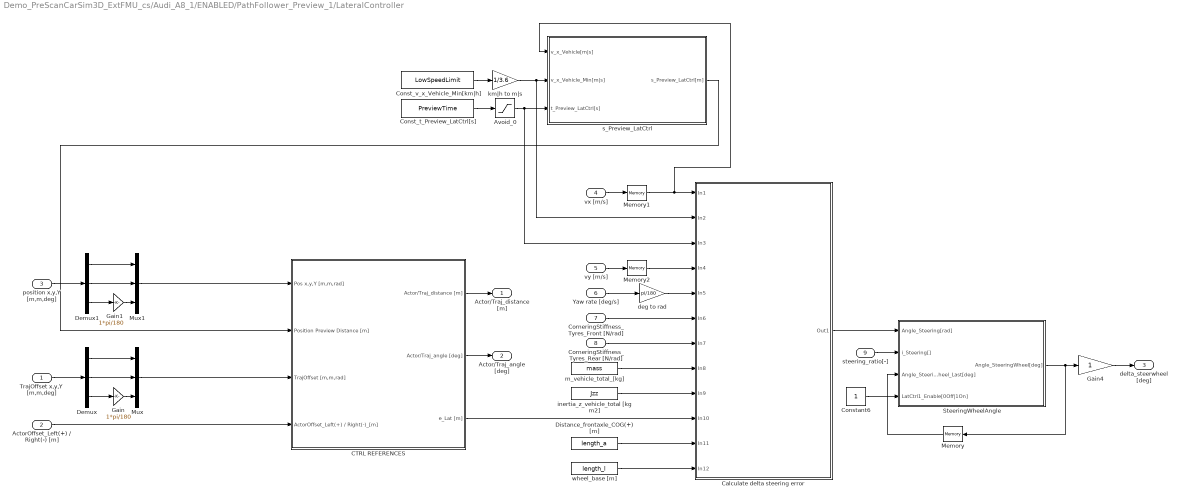
== system Demo_PreScanCarSim3D_ExtFMU_cs/Audi_A8_1/ENABLED/PathFollower_Preview_1/LateralController ==
  TrajOffset x,y,Y [m,m,deg] : Inport
  ActorOffset_Left(+) / Right(-) [m] : Inport  Port=2
  position x,y,Y [m,m,deg] : Inport  Port=3
  vx [m/s] : Inport  Port=4
  vy [m/s] : Inport  Port=5
  Yaw rate [deg/s] : Inport  Port=6
  CorneringStiffness_Tyres_Front [N/rad] : Inport  Port=7
  CorneringStiffness_Tyres_Rear [N/rad] : Inport  Port=8
  steering_ratio[-] : Inport  Port=9
  Avoid_0 : Saturate  UpperLimit=1000  LowerLimit=0.1
  CTRL REFERENCES : Subsystem
  Calculate delta steering error : Subsystem
      mask Display:
      | port_label('input', 1, 'v_x_vehicle [m/s]')
      | port_label('input', 2, 'v_x_vehicle_Min [m/s]')
      | port_label('input', 3, 't_Preview_LatCtrl [s]')
      | port_label('input', 4, 'v_y_vehicle [m/s]')
      | port_label('input', 5, 'yawrate_vehicle [rad/sec]')
      | port_label('input', 6, 'CorneringStiffness_Tyres_Front [N/rad]')
      | port_label('input', 7, 'CorneringStiffness_Tyres_Rear [N/rad]')
      | port_label('input', 8, 'm_vehicle_total [kg]')
      | port_label('input', 9, 'inertia_z_vehicle_total [kg m2]')
      | port_label('input', 10, 'e_Lat [m]')
      | port_label('input', 11, 'Distance_frontaxle_COG(+) [m]')
      | port_label('input', 12, 'wheel_base [m]')
      | port_label('output', 1, 'delta_steeringwheel [rad]')
  Const_t_Preview_LatCtrl[s] : Constant  Value=PreviewTime  SampleTime=CSSampleTime
  Const_v_x_Vehicle_Min[km|h] : Constant  Value=LowSpeedLimit  SampleTime=CSSampleTime
  Constant6 : Constant  SampleTime=CSSampleTime
  Demux : Demux  Outputs=3
  Demux1 : Demux  Outputs=3
  Distance_frontaxle_COG(+) [m] : Constant  Value=length_a  SampleTime=CSSampleTime
  Gain : Gain  Gain=1*pi/180
  Gain1 : Gain  Gain=1*pi/180
  Gain4 : Gain
  Memory : Memory  InheritSampleTime=on
  Memory1 : Memory  InheritSampleTime=on
  Memory2 : Memory  InheritSampleTime=on
  Mux : Mux  Inputs=3
  Mux1 : Mux  Inputs=3
  SteeringWheelAngle : Subsystem
  deg to rad : Gain  Gain=pi/180
  inertia_z_vehicle_total [kg m2] : Constant  Value=Jzz  SampleTime=CSSampleTime
  km|h to m|s : Gain  Gain=1/3.6
  m_vehicle_total_[kg] : Constant  Value=mass  SampleTime=CSSampleTime
  s_Preview_LatCtrl : Subsystem
  wheel_base [m] : Constant  Value=length_l  SampleTime=CSSampleTime
  Actor/Traj_distance [m] : Outport
  Actor/Traj_angle [deg] : Outport  Port=2
  delta_steerwheel [deg] : Outport  Port=3
  wires:
  km|h to m|s/1 -> Calculate delta steering error/2(In2), s_Preview_LatCtrl/2(v_x_Vehicle_Min[m|s])
  Gain/1 -> Mux/3
  Mux/1 -> CTRL REFERENCES/3(TrajOffset [m,m,rad])
  ActorOffset_Left(+) / Right(-) [m]/1 -> CTRL REFERENCES/4(ActorOffset_Left(+) / Right(-)_[m])
  Demux/1 -> Mux/1
  Demux/2 -> Mux/2
  Demux/3 -> Gain/1
  TrajOffset x,y,Y [m,m,deg]/1 -> Demux/1
  CTRL REFERENCES/2(Actor/Traj_angle [deg]) -> Actor/Traj_angle [deg]/1
  CTRL REFERENCES/1(Actor/Traj_distance [m]) -> Actor/Traj_distance [m]/1
  Calculate delta steering error/1(Out1) -> SteeringWheelAngle/1(Angle_Steering[rad])
  vx [m/s]/1 -> Memory1/1
  vy [m/s]/1 -> Memory2/1
  CorneringStiffness_Tyres_Front [N/rad]/1 -> Calculate delta steering error/6(In6)
  m_vehicle_total_[kg]/1 -> Calculate delta steering error/8(In8)
  inertia_z_vehicle_total [kg m2]/1 -> Calculate delta steering error/9(In9)
  steering_ratio[-]/1 -> SteeringWheelAngle/2(i_Steering[])
  SteeringWheelAngle/1(Angle_SteeringWheel[deg]) -> Gain4/1, Memory/1
  Memory/1 -> SteeringWheelAngle/3(Angle_SteeringWheel_Last[deg])
  Constant6/1 -> SteeringWheelAngle/4(LatCtrl1_Enable[0Off|1On])
  Avoid_0/1 -> Calculate delta steering error/3(In3), s_Preview_LatCtrl/3(t_Preview_LatCtrl[s])
  Const_v_x_Vehicle_Min[km|h]/1 -> km|h to m|s/1
  s_Preview_LatCtrl/1(s_Preview_LatCtrl[m]) -> CTRL REFERENCES/2(Position Preview Distance [m])
  Const_t_Preview_LatCtrl[s]/1 -> Avoid_0/1
  Gain4/1 -> delta_steerwheel [deg]/1
  Distance_frontaxle_COG(+) [m]/1 -> Calculate delta steering error/11(In11)
  CorneringStiffness_Tyres_Rear [N/rad]/1 -> Calculate delta steering error/7(In7)
  Yaw rate [deg/s]/1 -> deg to rad/1
  deg to rad/1 -> Calculate delta steering error/5(In5)
  Gain1/1 -> Mux1/3
  Demux1/1 -> Mux1/1
  Demux1/2 -> Mux1/2
  Demux1/3 -> Gain1/1
  position x,y,Y [m,m,deg]/1 -> Demux1/1
  Mux1/1 -> CTRL REFERENCES/1(Pos x,y,Y [m,m,rad])
  wheel_base [m]/1 -> Calculate delta steering error/12(In12)
  CTRL REFERENCES/3(e_Lat [m]) -> Calculate delta steering error/10(In10)
  Memory1/1 -> Calculate delta steering error/1(In1), s_Preview_LatCtrl/1(v_x_Vehicle[m|s])
  Memory2/1 -> Calculate delta steering error/4(In4)

== system Demo_PreScanCarSim3D_ExtFMU_cs/Audi_A8_1/ENABLED/PathFollower_Preview_1/LongitudinalController ==
  v_actual [m/s] : Inport
  Desired Velocity [m/s] : Inport  Port=2
  Initial Velocity [m/s] : Inport  Port=3
  Check_Initial_Velocity : Subsystem
  Demux : Demux  Outputs=3
  GearNormal : Constant
  "GearNormal " : Constant
  If Desired Velocity = 0 : Subsystem  TreatAsAtomicUnit=on
  If Desired Velocity ~= 0 : Subsystem  TreatAsAtomicUnit=on
  Memory External IC : Subsystem
  Merge : Merge
  Mux : Mux  Inputs=3
  Mux2 : Mux  Inputs=3
  Sum4 : Sum  Inputs=|+-
  if : If  IfExpression=u1 == 0  SampleTime=CSSampleTime
  throttle [%] : Outport
  brake pressure [bar] : Outport  Port=2
  v0 [m/s] : Outport  Port=3
  Auto_GearShift : Outport  Port=4
  wires:
  v_actual [m/s]/1 -> Check_Initial_Velocity/1(" v_actual_[m|s]"), Memory External IC/1(u)
  Memory External IC/1(y) -> Sum4/2
  Sum4/1 -> If Desired Velocity ~= 0/2(Desired Velocity [m/s])
  Desired Velocity [m/s]/1 -> if/1, Sum4/1
  Initial Velocity [m/s]/1 -> Check_Initial_Velocity/2(Initial_Velocity_[m|s]), Memory External IC/2(IC), v0 [m/s]/1
  GearNormal/1 -> If Desired Velocity = 0/1(In1)
  Merge/1 -> Demux/1
  If Desired Velocity = 0/1(throttle [%]) -> Mux/1
  If Desired Velocity = 0/2(brake pressure [bar]) -> Mux/2
  Mux2/1 -> Merge/2
  Mux/1 -> Merge/1
  Demux/1 -> throttle [%]/1
  Demux/2 -> brake pressure [bar]/1
  Demux/3 -> Auto_GearShift/1
  "GearNormal "/1 -> If Desired Velocity ~= 0/1(In1)
  If Desired Velocity = 0/3(Auto_GearShift) -> Mux/3
  if/2 -> If Desired Velocity ~= 0/Action
  if/1 -> If Desired Velocity = 0/Action
  If Desired Velocity ~= 0/1(throttle [%]) -> Mux2/1
  If Desired Velocity ~= 0/2(brake pressure [bar]) -> Mux2/2
  If Desired Velocity ~= 0/3(Auto_GearShift) -> Mux2/3

== system Demo_PreScanCarSim3D_ExtFMU_cs/Audi_A8_1/ENABLED/PreScan_RayCast_Contact_Sensor/Contact Point Bus Creator ==
  demux in : Inport
  Bus Creator : BusCreator  Inputs=3
  Bus Creator1 : BusCreator  Inputs=3
  Bus Creator2 : BusCreator  Inputs=3
  Demux : Demux  Outputs=3
  Demux5 : Demux  Outputs=[3 3 1]
  Demux6 : Demux  Outputs=3
  bus out : Outport
  wires:
  Demux/1 -> Bus Creator/1  "x"
  Demux/2 -> Bus Creator/2  "y"
  Demux/3 -> Bus Creator/3  "z"
  Demux6/1 -> Bus Creator1/1  "x"
  Demux6/2 -> Bus Creator1/2  "y"
  Demux6/3 -> Bus Creator1/3  "z"
  demux in/1 -> Demux5/1
  Demux5/3 -> Bus Creator2/3  "penetrationdepth"
  Bus Creator2/1 -> bus out/1
  Demux5/1 -> Demux/1
  Demux5/2 -> Demux6/1
  Bus Creator/1 -> Bus Creator2/1  "normal"
  Bus Creator1/1 -> Bus Creator2/2  "position"

== system Demo_PreScanCarSim3D_ExtFMU_cs/Audi_A8_1/ENABLED/PreScan_RayCast_Contact_Sensor/Contact Point Bus Creator1 ==
  demux in : Inport
  Bus Creator : BusCreator  Inputs=3
  Bus Creator1 : BusCreator  Inputs=3
  Bus Creator2 : BusCreator  Inputs=3
  Demux : Demux  Outputs=3
  Demux5 : Demux  Outputs=[3 3 1]
  Demux6 : Demux  Outputs=3
  bus out : Outport
  wires:
  Bus Creator1/1 -> Bus Creator2/2  "position"
  Bus Creator/1 -> Bus Creator2/1  "normal"
  Demux5/2 -> Demux6/1
  Demux5/1 -> Demux/1
  Bus Creator2/1 -> bus out/1
  Demux5/3 -> Bus Creator2/3  "penetrationdepth"
  demux in/1 -> Demux5/1
  Demux6/3 -> Bus Creator1/3  "z"
  Demux6/2 -> Bus Creator1/2  "y"
  Demux6/1 -> Bus Creator1/1  "x"
  Demux/3 -> Bus Creator/3  "z"
  Demux/2 -> Bus Creator/2  "y"
  Demux/1 -> Bus Creator/1  "x"

== system Demo_PreScanCarSim3D_ExtFMU_cs/Audi_A8_1/ENABLED/PreScan_RayCast_Contact_Sensor/Contact Point Bus Creator2 ==
  demux in : Inport
  Bus Creator : BusCreator  Inputs=3
  Bus Creator1 : BusCreator  Inputs=3
  Bus Creator2 : BusCreator  Inputs=3
  Demux : Demux  Outputs=3
  Demux5 : Demux  Outputs=[3 3 1]
  Demux6 : Demux  Outputs=3
  bus out : Outport
  wires:
  Bus Creator1/1 -> Bus Creator2/2  "position"
  Bus Creator/1 -> Bus Creator2/1  "normal"
  Demux5/2 -> Demux6/1
  Demux5/1 -> Demux/1
  Bus Creator2/1 -> bus out/1
  Demux5/3 -> Bus Creator2/3  "penetrationdepth"
  demux in/1 -> Demux5/1
  Demux6/3 -> Bus Creator1/3  "z"
  Demux6/2 -> Bus Creator1/2  "y"
  Demux6/1 -> Bus Creator1/1  "x"
  Demux/3 -> Bus Creator/3  "z"
  Demux/2 -> Bus Creator/2  "y"
  Demux/1 -> Bus Creator/1  "x"

== system Demo_PreScanCarSim3D_ExtFMU_cs/Audi_A8_1/ENABLED/PreScan_RayCast_Contact_Sensor/Contact Point Bus Creator3 ==
  demux in : Inport
  Bus Creator : BusCreator  Inputs=3
  Bus Creator1 : BusCreator  Inputs=3
  Bus Creator2 : BusCreator  Inputs=3
  Demux : Demux  Outputs=3
  Demux5 : Demux  Outputs=[3 3 1]
  Demux6 : Demux  Outputs=3
  bus out : Outport
  wires:
  Bus Creator1/1 -> Bus Creator2/2  "position"
  Bus Creator/1 -> Bus Creator2/1  "normal"
  Demux5/2 -> Demux6/1
  Demux5/1 -> Demux/1
  Bus Creator2/1 -> bus out/1
  Demux5/3 -> Bus Creator2/3  "penetrationdepth"
  demux in/1 -> Demux5/1
  Demux6/3 -> Bus Creator1/3  "z"
  Demux6/2 -> Bus Creator1/2  "y"
  Demux6/1 -> Bus Creator1/1  "x"
  Demux/3 -> Bus Creator/3  "z"
  Demux/2 -> Bus Creator/2  "y"
  Demux/1 -> Bus Creator/1  "x"
